simulink model "MassaMolaEstabilidade"  (Simulink 7.5)
settings: Solver=ode45  StartTime=0.0  StopTime=500  RelTol=1e-3
settings Model: Creator=Leonardo  LastModifiedBy=Leo

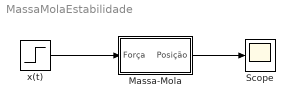
== system MassaMolaEstabilidade ==
  Massa-Mola : Subsystem
  Scope : Scope
  x(t) : Step  Time=0  After=20  SampleTime=0
  wires:
  x(t)/1 -> Massa-Mola/1(Força)
  Massa-Mola/1(Posição) -> Scope/1

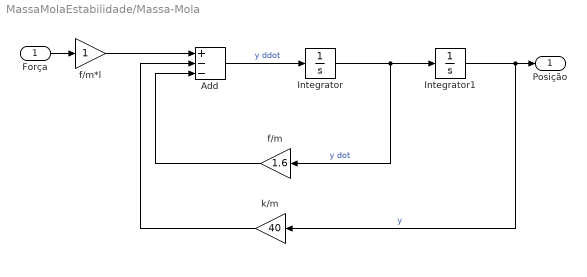
== system MassaMolaEstabilidade/Massa-Mola ==
  Força : Inport
  Add : Sum  Inputs=+--
  Integrator : Integrator
  Integrator1 : Integrator
  f/m : Gain  Gain=1.6
  f/m*l : Gain
  k/m : Gain  Gain=40
  Posição : Outport
  wires:
  Integrator/1 -> Integrator1/1, f/m/1  "y dot"
  Add/1 -> Integrator/1  "y ddot"
  Integrator1/1 -> Posição/1, k/m/1  "y"
  k/m/1 -> Add/2
  f/m/1 -> Add/3
  f/m*l/1 -> Add/1
  Força/1 -> f/m*l/1
